simulink model "pH_successive_Linearization_new"  (R2021a)
settings: Solver=ode15s  StartTime=0.0  StopTime=3000  RelTol=1e-3
undefined symbols (not defined in the file or in its folder): sigbuilder_block
libraries: mpclib x1, simulink x1
settings Model: Creator=NIFEMI  LastModifiedBy=USER
settings SolverCC: AlgebraicLoopSolver=TrustRegion
settings DataIOCC: ReturnWorkspaceOutputs=off
settings DebuggingCC: PregeneratedLibrarySubsystemCodeDiagnostic=none  SFMachineParentedDataDiag=warning  ArithmeticOperatorsInVariantConditions=warning
settings SFSimCC: CustomCodeUndefinedFunction=UseInterfaceOnly

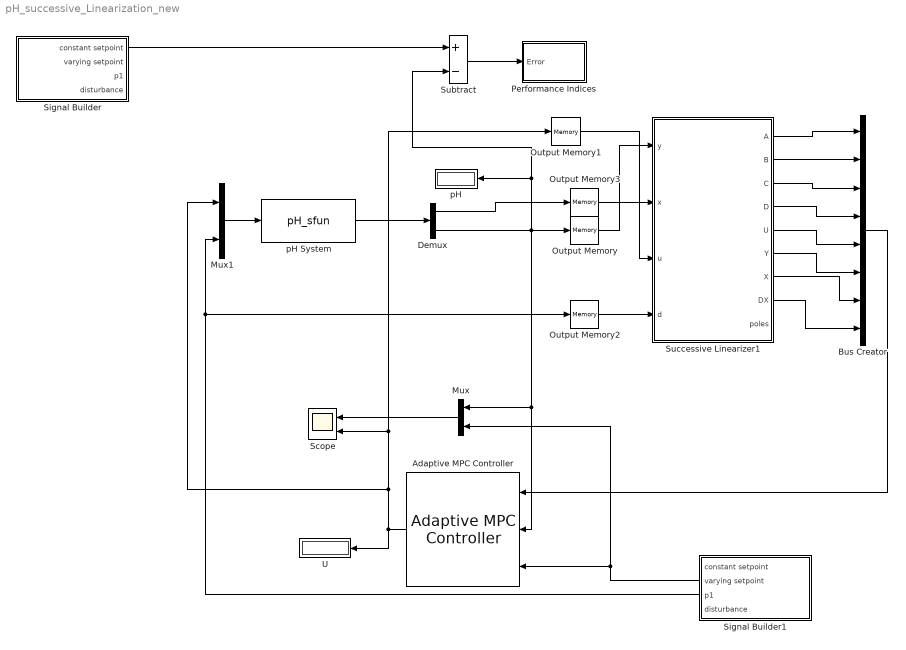
== system pH_successive_Linearization_new ==
  Adaptive MPC Controller : mpclib/Adaptive MPC Controller  SCDEnableBlockLinearizationSpecification=on  mpcobj=mpcobj_sl  enable_value=0  updateMPCinCallerWorkspace=on  md_inport=off  mv_inport=off  uref_inport=off  return_cost=off  return_mvseq=off  return_qpstatus=off  return_xseq=off  return_state=off  return_ovseq=off  state_inport=off  isltv_plant=off  umin_inport=off  umax_inport=off  ymin_inport=off  ymax_inport=off  cc_inport=off  ywt_inport=off  uwt_inport=off  duwt_inport=off  rhoeps_inport=off  pm_inport=off  MaximumP=10  HorizonChoice=FixedHorizon  BlockDataType=double  SampleTimeInherited=off  switch_inport=off
  Bus Creator : BusCreator  Inputs=8
  Demux : Demux  Outputs=2
  Mux : Mux  Inputs=2
  Mux1 : Mux  Inputs=2
  Output Memory : Memory  InitialCondition=2.542
  Output Memory1 : Memory  InitialCondition=0.8
  Output Memory2 : Memory  InitialCondition=13
  Output Memory3 : Memory  InitialCondition=0.13
  Performance Indices : Subsystem
  Scope : Scope  NumInputPorts=2
  Signal Builder : Subsystem  Tag=STV Subsys  LoadFcn=sigbuilder_block('load');  StartFcn=sigbuilder_block('start');  StopFcn=sigbuilder_block('stop');  ClipboardFcn=sigbuilder_block('clipboard');  mask(Sigbuilder block){tuvar=[0:10]}
      mask help: Simulink:masks:SigbuilderBlock_MD
      mask init:
      | if ~strcmp(get_param(bdroot(gcbh),'SimulationStatus'),'stopped') tuvar = sigbuilder_block('maskInit'); end
      settings: CopyFcn=sigbuilder_block('copy');  DeleteFcn=sigbuilder_block('delete');  ModelCloseFcn=sigbuilder_block('modelClose');  PreSaveFcn=sigbuilder_block('preSave');  PauseFcn=sigbuilder_block('pause');  ContinueFcn=sigbuilder_block('continue');  NameChangeFcn=sigbuilder_block('namechange');  OpenFcn=sigbuilder_block('open',[404 117.5 550.5 362.5 ]);  CloseFcn=sigbuilder_block('close');
      mask Display: plot(0, 0, 100, 100,[2, 2, 32, 32, 2], [68, 8, 8, 68, 68],[32, 2], [38, 38], [32, 19, 2],[53, 60, 44], [32, 17, 17, 2],[16, 16, 31, 31]);txt = getActiveGroup(gcbh);text(2, 100, txt,'verticalAlignment', 'top');
  Signal Builder1 : Subsystem  Tag=STV Subsys  LoadFcn=sigbuilder_block('load');  StartFcn=sigbuilder_block('start');  StopFcn=sigbuilder_block('stop');  ClipboardFcn=sigbuilder_block('clipboard');  mask(Sigbuilder block){tuvar=[0:10]}
      mask help: Simulink:masks:SigbuilderBlock_MD
      mask init:
      | if ~strcmp(get_param(bdroot(gcbh),'SimulationStatus'),'stopped') tuvar = sigbuilder_block('maskInit'); end
      settings: CopyFcn=sigbuilder_block('copy');  DeleteFcn=sigbuilder_block('delete');  ModelCloseFcn=sigbuilder_block('modelClose');  PreSaveFcn=sigbuilder_block('preSave');  PauseFcn=sigbuilder_block('pause');  ContinueFcn=sigbuilder_block('continue');  NameChangeFcn=sigbuilder_block('namechange');  OpenFcn=sigbuilder_block('open',[404 117.5 550.5 362.5 ]);  CloseFcn=sigbuilder_block('close');
      mask Display: plot(0, 0, 100, 100,[2, 2, 32, 32, 2], [68, 8, 8, 68, 68],[32, 2], [38, 38], [32, 19, 2],[53, 60, 44], [32, 17, 17, 2],[16, 16, 31, 31]);txt = getActiveGroup(gcbh);text(2, 100, txt,'verticalAlignment', 'top');
  Subtract : Sum  Inputs=+-
  Successive Linearizer1 : MATLAB Function  TreatAsAtomicUnit=on  SystemSampleTime=0.5
  U : Display
  pH : Display
  pH System : S-Function  FunctionName=pH_sfun  SFunctionDeploymentMode=off  EnableBusSupport=off
  wires:
  Successive Linearizer1/1(A) -> Bus Creator/1
  Successive Linearizer1/2(B) -> Bus Creator/2
  Successive Linearizer1/3(C) -> Bus Creator/3
  Successive Linearizer1/5(U) -> Bus Creator/5
  Successive Linearizer1/6(Y) -> Bus Creator/6
  Successive Linearizer1/7(X) -> Bus Creator/7
  Successive Linearizer1/8(DX) -> Bus Creator/8
  Successive Linearizer1/4(D) -> Bus Creator/4
  Bus Creator/1 -> Adaptive MPC Controller/1
  Mux/1 -> Scope/1
  Output Memory1/1 -> Successive Linearizer1/3(u)
  Subtract/1 -> Performance Indices/1(Error)
  Demux/2 -> Subtract/2, pH/1, Output Memory/1, Adaptive MPC Controller/2, Mux/1
  Signal Builder/1(constant setpoint) -> Subtract/1
  Signal Builder1/3(p1) -> Mux1/2, Output Memory2/1
  Adaptive MPC Controller/1 -> Mux1/1, Scope/2, Output Memory1/1, U/1
  Mux1/1 -> pH System/1
  Output Memory2/1 -> Successive Linearizer1/4(d)
  pH System/1 -> Demux/1
  Signal Builder1/2(varying setpoint) -> Mux/2, Adaptive MPC Controller/3
  Output Memory/1 -> Successive Linearizer1/1(y)
  Demux/1 -> Output Memory3/1
  Output Memory3/1 -> Successive Linearizer1/2(x)

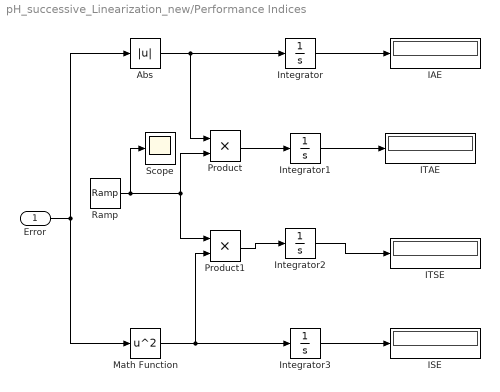
== system pH_successive_Linearization_new/Performance Indices ==
  Error : Inport
  Abs : Abs
  IAE : Display
  ISE : Display
  ITAE : Display
  ITSE : Display
  Integrator{,1..3} (4 alike) : Integrator
  Math Function : Math  Operator=square  SignedPower=on  SaturateOnIntegerOverflow=on
  Product : Product  RndMeth=Zero
  Product1 : Product  RndMeth=Zero
  Ramp : simulink/Sources/Ramp  slope=1  start=0  InitialOutput=0
  Scope : Scope
  wires:
  Error/1 -> Math Function/1, Abs/1
  Abs/1 -> Integrator/1, Product/1
  Integrator/1 -> IAE/1
  Ramp/1 -> Product/2, Product1/1, Scope/1
  Math Function/1 -> Integrator3/1, Product1/2
  Product1/1 -> Integrator2/1
  Product/1 -> Integrator1/1
  Integrator3/1 -> ISE/1
  Integrator2/1 -> ITSE/1
  Integrator1/1 -> ITAE/1

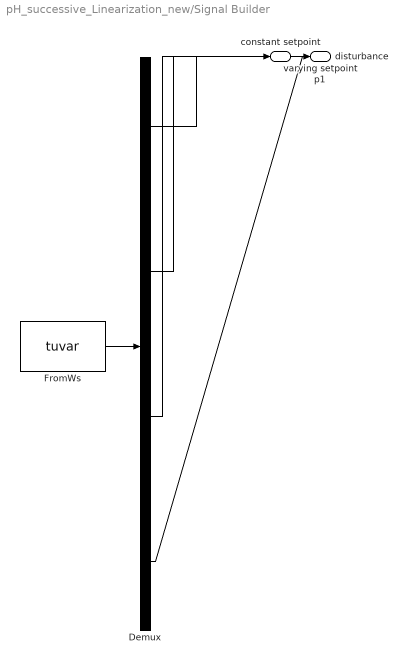
== system pH_successive_Linearization_new/Signal Builder ==
  Demux : Demux  Tag=STV Demux
      settings: DisplayOption=none
  FromWs : FromWorkspace  Tag=STV FromWs  VariableName=tuvar
      SigBuilderData=|
      | common.afterFinalStr = 'Extrapolate'
      | common.sampleTime = 0
      | dataSet.timeRange = [0 3000]
      | dataSet.name = 'Group 1'
      | sbobj.Groups.Name = 'Group 1'
      | sbobj.Groups.Signals(1).Name = 'constant setpoint'
      | sbobj.Groups.Signals(1).XData = [0 3000]
      | sbobj.Groups.Signals(1).YData = [7 7]
      | sbobj.Groups.Signals(2).Name = 'varying setpoint'
      | sbobj.Groups.Signals(2).XData = [0 1000 1000 2000 2000 3000]
      | sbobj.Groups.Signals(2).YData = [2.95 2.95 10 10 6 6]
      | sbobj.Groups.Signals(3).Name = 'p1'
      | sbobj.Groups.Signals(3).XData = [0 3000]
      | sbobj.Groups.Signals(3).YData = [13 13]
      | sbobj.Groups.Signals(4).Name = 'disturbance'
      | sbobj.Groups.Signals(4).XData = [0 495 495 1000 1000 1500 1500 1995 1995 2495 2495 3000]
      | sbobj.Groups.Signals(4).YData = [13 13 15 15 13 13 10 10 13 13 15 15]
      | sbobj.Groups.TimeRange = [0 3000]
  constant setpoint : Outport  Tag=STV Outport
  varying setpoint : Outport  Tag=STV Outport  Port=2
  p1 : Outport  Tag=STV Outport  Port=3
  disturbance : Outport  Tag=STV Outport  Port=4
  wires:
  Demux/1 -> constant setpoint/1
  FromWs/1 -> Demux/1
  Demux/2 -> varying setpoint/1
  Demux/3 -> p1/1
  Demux/4 -> disturbance/1

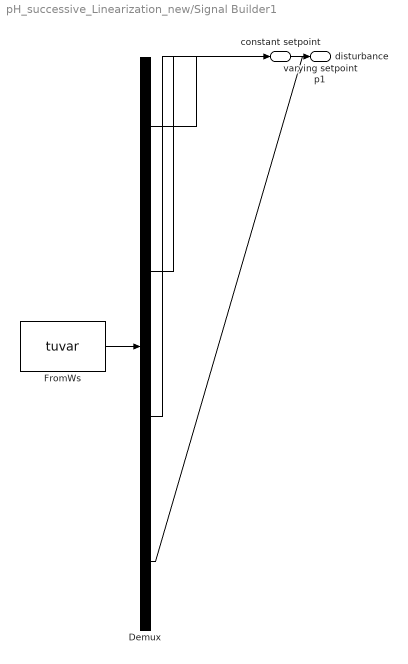
== system pH_successive_Linearization_new/Signal Builder1 ==
  Demux : Demux  Tag=STV Demux
      settings: DisplayOption=none
  FromWs : FromWorkspace  Tag=STV FromWs  VariableName=tuvar
      SigBuilderData=|
      | common.afterFinalStr = 'Extrapolate'
      | common.sampleTime = 0
      | dataSet.timeRange = [0 3000]
      | dataSet.name = 'Group 1'
      | sbobj.Groups.Name = 'Group 1'
      | sbobj.Groups.Signals(1).Name = 'constant setpoint'
      | sbobj.Groups.Signals(1).XData = [0 3000]
      | sbobj.Groups.Signals(1).YData = [7 7]
      | sbobj.Groups.Signals(2).Name = 'varying setpoint'
      | sbobj.Groups.Signals(2).XData = [0 1000 1000 2000 2000 3000]
      | sbobj.Groups.Signals(2).YData = [2.95 2.95 10 10 6 6]
      | sbobj.Groups.Signals(3).Name = 'p1'
      | sbobj.Groups.Signals(3).XData = [0 3000]
      | sbobj.Groups.Signals(3).YData = [13 13]
      | sbobj.Groups.Signals(4).Name = 'disturbance'
      | sbobj.Groups.Signals(4).XData = [0 495 495 1000 1000 1500 1500 1995 1995 2495 2495 3000]
      | sbobj.Groups.Signals(4).YData = [13 13 15 15 13 13 10 10 13 13 15 15]
      | sbobj.Groups.TimeRange = [0 3000]
  constant setpoint : Outport  Tag=STV Outport
  varying setpoint : Outport  Tag=STV Outport  Port=2
  p1 : Outport  Tag=STV Outport  Port=3
  disturbance : Outport  Tag=STV Outport  Port=4
  wires:
  Demux/1 -> constant setpoint/1
  FromWs/1 -> Demux/1
  Demux/2 -> varying setpoint/1
  Demux/3 -> p1/1
  Demux/4 -> disturbance/1

== matlab function pH_successive_Linearization_new/Successive Linearizer1 ==
  data: y input size=[1,1]; x input; u input; A output size=[1,1]; B output size=[1 1]; C output size=[1,1]; D output size=[1 1]; U output size=[1,1]; Y output size=[1,1]; X output size=[1,1]; DX output size=[1,1]; d input; poles output
function [A, B, C, D, U, Y, X, DX,poles] = fcn(y, x, u, d)

%%%%%%%%%%%%%%%%%%%%%%%%%%%%%%%%%%%%%%%%%%%%%%%%%%%%%%%
%#codegen

% Define constant outputs
Ts = 0.3;
U = u(1) ;
Y = y ;
X = x(1);

% Analytical linearization of mechanistic CSTR model (continuous time)
% [A, Bo] = getContinuous(T, CA, CAi, Ti, Tc);
[a, b, c, d] = getContinuous(y, x, u, d, Ts)  ;

% Convert continuous to discrete time
% [A, Bo] = getDiscrete(A, Bo, Ts);
[A, Bo, C, D] = getDiscrete(a, b, c, d, Ts)   ;
% Last column of B contains the constant offset contribution.
DX = 0;%Bo(:,2);
B = Bo(:,1);
% Compute poles
poles = abs(eig(A));

end

%%%%%%%%%%%%%%%%%%%%%%%%%%%%%%%%%%%%%%%%%%%%%%%%%%%%%
%%%%%%%%%%%%%%%%%%%%%%%%%%%%%%%%%%%

function [a, b, c, d] = getContinuous(y, x, u, d, Ts)




% [A, B, C, D] = get_discrete_model(y, x, u, d, Ts)   ;

%%%%%%%%%%%%%%%%%%%%%%%%%%%%%%%%%%%%%
    m = u(1);
      F = d(1);
      N = x(1);
      
      p2 = 0.001;
      p3 = 0.13;
%    
      dNdt = 0.0111*(m-(F+m)*N);
       dxdt = dNdt;
       x1 = N;
        f = [1,(p2 + x1),(x1*p2 -10^(-14) -p2*p3),-(10^(-14)*p2)]  ;
        x2 = max(roots(f)) ;
       

    %%%%%%%%%%%%%%%%%%%%%%%%%%%%%%%%%%

    pH = y(1);   
    
a = - (111*F)/10000 - (111*m)/10000;
b = 111/10000 - (111*N)/10000;
c = (p2/10^pH + 1/10^(2*pH))/(3/10^(3*pH)*log(10) - (log(10)*(p2*p3 - N*p2 + 1/100000000000000))/10^pH + 2/10^(2*pH)*log(10)*(N + p2));
d = 0;     

end


function [A, B, C, D] = getDiscrete(a, b,c,d, Ts)
% Convert to discrete time
A = expm(a*Ts);
nx = size(b,1);
n = 4;  % Number of points for Simpson's Rule, an even integer >= 2.
% Use Simpson's rule to compute integral(0,Ts){expm(a*s)*ds*b}
h = Ts/n;
Ai = eye(nx) + A;        % First and last terms;
Coef = 2;
for i = 1:n-1
    if Coef == 2
        Coef = 4;
    else
        Coef = 2;
    end
    Ai = Ai + Coef*expm(a*i*h);     % Intermediate terms
end
B = (h/3)*Ai*b;

C = c  ;
D = d ;
end
